simulink model "model_4_1"  (R2021a)
settings: Solver=VariableStepAuto  StartTime=0.0  StopTime=300  RelTol=1e-3
settings Model: Creator=alamg  LastModifiedBy=alamg

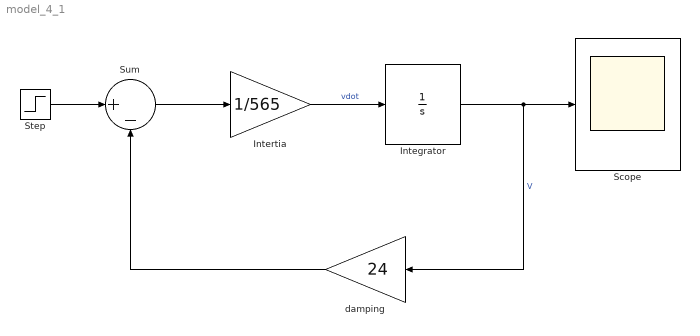
== system model_4_1 ==
  Integrator : Integrator
  Intertia : Gain  Gain=1/565
  Scope : Scope
  Step : Step  Time=0.2  After=1000  SampleTime=0
  Sum : Sum  Inputs=|+-
  damping : Gain  Gain=24
  wires:
  Integrator/1 -> damping/1, Scope/1  "V"
  Intertia/1 -> Integrator/1  "vdot"
  Sum/1 -> Intertia/1
  damping/1 -> Sum/2
  Step/1 -> Sum/1
